simulink model "CounterLab"  (R2022b)
settings: Solver=FixedStepAuto  StartTime=0.0  StopTime=10  FixedStep=1e-3  RelTol=1e-3
libraries: simulink x1
settings Model: Creator=ahmed  LastModifiedBy=ahmed

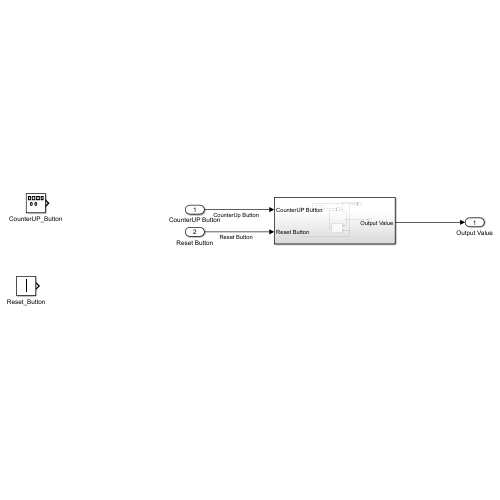
[thumbnail: Simulink's stored preview of the top-level diagram]
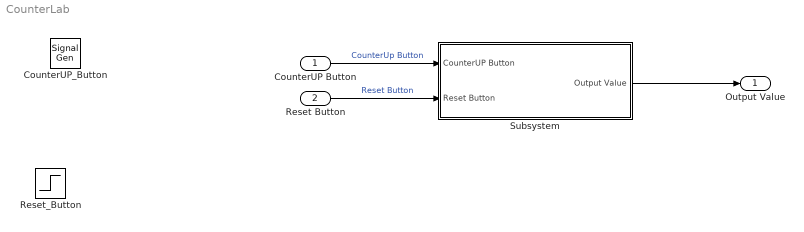
== system CounterLab ==
  CounterUP Button : Inport
  Reset Button : Inport  Port=2
  CounterUP_Button : SignalGenerator  WaveForm=square
  Reset_Button : Step  Time=5  SampleTime=0
  Subsystem : Subsystem
  Output Value : Outport
  wires:
  CounterUP Button/1 -> Subsystem/1(CounterUP Button)  "CounterUp Button"
  Reset Button/1 -> Subsystem/2(Reset Button)  "Reset Button"
  Subsystem/1(Output Value) -> Output Value/1

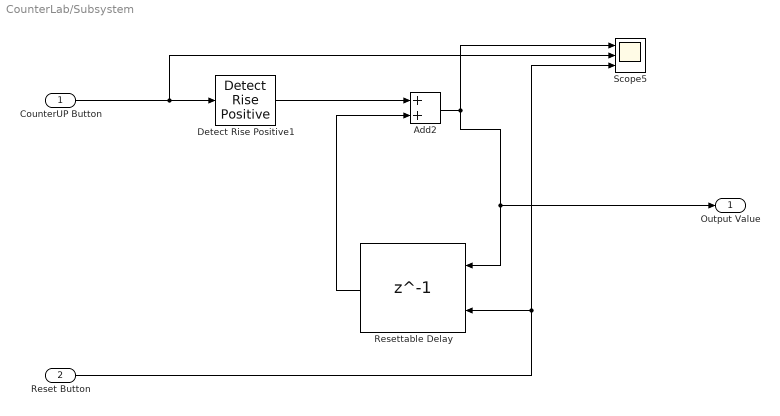
== system CounterLab/Subsystem ==
  CounterUP Button : Inport
  Reset Button : Inport  Port=2
  Add2 : Sum
  Detect Rise Positive1 : simulink/Logic and Bit Operations/Detect Rise Positive  vinit=0  OutDataTypeStr=uint8
  Resettable Delay : Delay  DelayLength=1  ExternalReset=Rising
      settings: InputPortMap=u0,r5
  Scope5 : Scope  NumInputPorts=3
  Output Value : Outport
  wires:
  CounterUP Button/1 -> Scope5/2, Detect Rise Positive1/1
  Resettable Delay/1 -> Add2/2
  Reset Button/1 -> Scope5/3, Resettable Delay/2
  Add2/1 -> Output Value/1, Resettable Delay/1, Scope5/1
  Detect Rise Positive1/1 -> Add2/1
